simulink model "angle_controller"  (R2015a)
settings: Solver=ode45  StartTime=0.0  StopTime=20  RelTol=1e-3
libraries: cstblocks x2, simulink x1
settings Model: Creator=morten  LastModifiedBy=morten

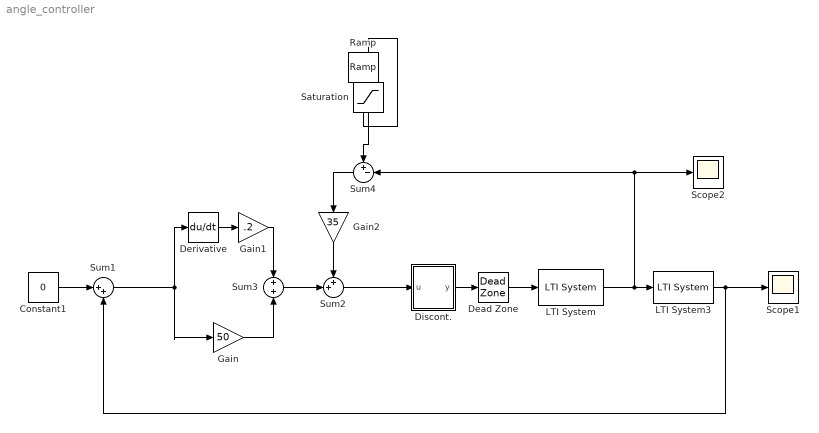
== system angle_controller ==
  Constant1 : Constant  Value=0
  Dead Zone : DeadZone  LowerValue=-4.5  UpperValue=4.5  SaturateOnIntegerOverflow=on
  Derivative : Derivative
  Discont. : MATLAB Function  TreatAsAtomicUnit=on
  Gain : Gain  Gain=50
  Gain1 : Gain  Gain=.2
  Gain2 : Gain  Gain=35
  LTI System : cstblocks/LTI System  sys=X  IC=[]
  LTI System3 : cstblocks/LTI System  sys=W  IC=[]
  Ramp : simulink/Sources/Ramp  slope=.75  start=0  X0=0
  Saturation : Saturate  UpperLimit=4  LowerLimit=0
  Scope1 : Scope
      settings: YMin=-2e-05  YMax=-3e-06
  Scope2 : Scope
  Sum1 : Sum  Inputs=|++
  Sum2 : Sum  Inputs=++|
  Sum3 : Sum  Inputs=+|+
  Sum4 : Sum  Inputs=+-|
  wires:
  LTI System/1 -> Sum4/2, Scope2/1, LTI System3/1
  Constant1/1 -> Sum1/1
  LTI System3/1 -> Sum1/2, Scope1/1
  Sum2/1 -> Discont./1(u)
  Ramp/1 -> Saturation/1
  Saturation/1 -> Sum4/1
  Sum1/1 -> Derivative/1, Gain/1
  Derivative/1 -> Gain1/1
  Sum3/1 -> Sum2/2
  Sum4/1 -> Gain2/1
  Gain2/1 -> Sum2/1
  Gain/1 -> Sum3/2
  Discont./1(y) -> Dead Zone/1
  Dead Zone/1 -> LTI System/1
  Gain1/1 -> Sum3/1

== matlab function angle_controller/Discont. ==
  data: u input; y output
function y = dis(u)
    if(u > -4.6 && u < -0.2)
        y = -4.6;
    elseif(u < 4.6 && u > 0.2)
        y = 4.6;
    elseif( u < 0.2 && u > -0.2)
        y = 0;
    elseif(u > 12.5)
        y = 12.5;
    elseif(u < -12.5)
        y = -12.5;
    else
        y = u;
end
